simulink model "c00011M_harness"  (R2018a)
settings: Solver=FixedStepAuto  StartTime=0.0  StopTime=300  FixedStep=0.1  RelTol=1e-3
undefined symbols (not defined in the file): A1, hmax, PriorityTank, R1, R2, sigbuilder_block
(part 72 of 73)

== stateflow chart c00011M_harness/M160/Tank1/Control/Maintenance/Chart ==
  state InitialState
    entry: LiquidIn = 0;
    LiquidOut = 0;
  state Step1
    entry: LiquidIn = 0;
    LiquidOut = 1;
  state Step2
    entry: LiquidIn = 1;
    LiquidOut = 0;
  state Step3
    entry: LiquidIn = 0;
    LiquidOut = 1;
  (default) -> InitialState
  Step3 -> InitialState : [Type~=1||LiquidLevel <=0.01]
  Step2 -> InitialState [order 1] : [Type~=1]
  Step1 -> InitialState [order 1] : [Type ~= 1]
  InitialState -> Step1 : [StartMaintenance == 1 && Type ==1]
  Step1 -> Step2 [order 2] : [LiquidLevel <=0.01]
  Step2 -> Step3 [order 2] : [LiquidLevel>=hmax*0.9]
  data: Type input; StartMaintenance input; LiquidIn output; LiquidOut output; LiquidLevel input; hmax parameter

== stateflow chart c00011M_harness/M160/Tank2/Control/Maintenance/Chart ==
  state InitialState
    entry: LiquidIn = 0;
    LiquidOut = 0;
  state Step1
    entry: LiquidIn = 0;
    LiquidOut = 1;
  state Step2
    entry: LiquidIn = 1;
    LiquidOut = 0;
  state Step3
    entry: LiquidIn = 0;
    LiquidOut = 1;
  (default) -> InitialState
  Step3 -> InitialState : [Type~=1||LiquidLevel <=0.01]
  Step2 -> InitialState [order 1] : [Type~=1]
  Step1 -> InitialState [order 1] : [Type ~= 1]
  InitialState -> Step1 : [StartMaintenance == 1 && Type ==1]
  Step1 -> Step2 [order 2] : [LiquidLevel <=0.01]
  Step2 -> Step3 [order 2] : [LiquidLevel>=hmax*0.9]
  data: Type input; StartMaintenance input; LiquidIn output; LiquidOut output; LiquidLevel input; hmax parameter

== stateflow chart c00011M_harness/M161/Tank1/Control/Maintenance/Chart ==
  state InitialState
    entry: LiquidIn = 0;
    LiquidOut = 0;
  state Step1
    entry: LiquidIn = 0;
    LiquidOut = 1;
  state Step2
    entry: LiquidIn = 1;
    LiquidOut = 0;
  state Step3
    entry: LiquidIn = 0;
    LiquidOut = 1;
  (default) -> InitialState
  Step3 -> InitialState : [Type~=1||LiquidLevel <=0.01]
  Step2 -> InitialState [order 1] : [Type~=1]
  Step1 -> InitialState [order 1] : [Type ~= 1]
  InitialState -> Step1 : [StartMaintenance == 1 && Type ==1]
  Step1 -> Step2 [order 2] : [LiquidLevel <=0.01]
  Step2 -> Step3 [order 2] : [LiquidLevel>=hmax*0.9]
  data: Type input; StartMaintenance input; LiquidIn output; LiquidOut output; LiquidLevel input; hmax parameter

== stateflow chart c00011M_harness/M161/Tank2/Control/Maintenance/Chart ==
  state InitialState
    entry: LiquidIn = 0;
    LiquidOut = 0;
  state Step1
    entry: LiquidIn = 0;
    LiquidOut = 1;
  state Step2
    entry: LiquidIn = 1;
    LiquidOut = 0;
  state Step3
    entry: LiquidIn = 0;
    LiquidOut = 1;
  (default) -> InitialState
  Step3 -> InitialState : [Type~=1||LiquidLevel <=0.01]
  Step2 -> InitialState [order 1] : [Type~=1]
  Step1 -> InitialState [order 1] : [Type ~= 1]
  InitialState -> Step1 : [StartMaintenance == 1 && Type ==1]
  Step1 -> Step2 [order 2] : [LiquidLevel <=0.01]
  Step2 -> Step3 [order 2] : [LiquidLevel>=hmax*0.9]
  data: Type input; StartMaintenance input; LiquidIn output; LiquidOut output; LiquidLevel input; hmax parameter

== stateflow chart c00011M_harness/M162/Tank1/Control/Maintenance/Chart ==
  state InitialState
    entry: LiquidIn = 0;
    LiquidOut = 0;
  state Step1
    entry: LiquidIn = 0;
    LiquidOut = 1;
  state Step2
    entry: LiquidIn = 1;
    LiquidOut = 0;
  state Step3
    entry: LiquidIn = 0;
    LiquidOut = 1;
  (default) -> InitialState
  Step3 -> InitialState : [Type~=1||LiquidLevel <=0.01]
  Step2 -> InitialState [order 1] : [Type~=1]
  Step1 -> InitialState [order 1] : [Type ~= 1]
  InitialState -> Step1 : [StartMaintenance == 1 && Type ==1]
  Step1 -> Step2 [order 2] : [LiquidLevel <=0.01]
  Step2 -> Step3 [order 2] : [LiquidLevel>=hmax*0.9]
  data: Type input; StartMaintenance input; LiquidIn output; LiquidOut output; LiquidLevel input; hmax parameter

== stateflow chart c00011M_harness/M162/Tank2/Control/Maintenance/Chart ==
  state InitialState
    entry: LiquidIn = 0;
    LiquidOut = 0;
  state Step1
    entry: LiquidIn = 0;
    LiquidOut = 1;
  state Step2
    entry: LiquidIn = 1;
    LiquidOut = 0;
  state Step3
    entry: LiquidIn = 0;
    LiquidOut = 1;
  (default) -> InitialState
  Step3 -> InitialState : [Type~=1||LiquidLevel <=0.01]
  Step2 -> InitialState [order 1] : [Type~=1]
  Step1 -> InitialState [order 1] : [Type ~= 1]
  InitialState -> Step1 : [StartMaintenance == 1 && Type ==1]
  Step1 -> Step2 [order 2] : [LiquidLevel <=0.01]
  Step2 -> Step3 [order 2] : [LiquidLevel>=hmax*0.9]
  data: Type input; StartMaintenance input; LiquidIn output; LiquidOut output; LiquidLevel input; hmax parameter

== stateflow chart c00011M_harness/M163/Tank1/Control/Maintenance/Chart ==
  state InitialState
    entry: LiquidIn = 0;
    LiquidOut = 0;
  state Step1
    entry: LiquidIn = 0;
    LiquidOut = 1;
  state Step2
    entry: LiquidIn = 1;
    LiquidOut = 0;
  state Step3
    entry: LiquidIn = 0;
    LiquidOut = 1;
  (default) -> InitialState
  Step3 -> InitialState : [Type~=1||LiquidLevel <=0.01]
  Step2 -> InitialState [order 1] : [Type~=1]
  Step1 -> InitialState [order 1] : [Type ~= 1]
  InitialState -> Step1 : [StartMaintenance == 1 && Type ==1]
  Step1 -> Step2 [order 2] : [LiquidLevel <=0.01]
  Step2 -> Step3 [order 2] : [LiquidLevel>=hmax*0.9]
  data: Type input; StartMaintenance input; LiquidIn output; LiquidOut output; LiquidLevel input; hmax parameter

== stateflow chart c00011M_harness/M163/Tank2/Control/Maintenance/Chart ==
  state InitialState
    entry: LiquidIn = 0;
    LiquidOut = 0;
  state Step1
    entry: LiquidIn = 0;
    LiquidOut = 1;
  state Step2
    entry: LiquidIn = 1;
    LiquidOut = 0;
  state Step3
    entry: LiquidIn = 0;
    LiquidOut = 1;
  (default) -> InitialState
  Step3 -> InitialState : [Type~=1||LiquidLevel <=0.01]
  Step2 -> InitialState [order 1] : [Type~=1]
  Step1 -> InitialState [order 1] : [Type ~= 1]
  InitialState -> Step1 : [StartMaintenance == 1 && Type ==1]
  Step1 -> Step2 [order 2] : [LiquidLevel <=0.01]
  Step2 -> Step3 [order 2] : [LiquidLevel>=hmax*0.9]
  data: Type input; StartMaintenance input; LiquidIn output; LiquidOut output; LiquidLevel input; hmax parameter

== stateflow chart c00011M_harness/M164/Tank1/Control/Maintenance/Chart ==
  state InitialState
    entry: LiquidIn = 0;
    LiquidOut = 0;
  state Step1
    entry: LiquidIn = 0;
    LiquidOut = 1;
  state Step2
    entry: LiquidIn = 1;
    LiquidOut = 0;
  state Step3
    entry: LiquidIn = 0;
    LiquidOut = 1;
  (default) -> InitialState
  Step3 -> InitialState : [Type~=1||LiquidLevel <=0.01]
  Step2 -> InitialState [order 1] : [Type~=1]
  Step1 -> InitialState [order 1] : [Type ~= 1]
  InitialState -> Step1 : [StartMaintenance == 1 && Type ==1]
  Step1 -> Step2 [order 2] : [LiquidLevel <=0.01]
  Step2 -> Step3 [order 2] : [LiquidLevel>=hmax*0.9]
  data: Type input; StartMaintenance input; LiquidIn output; LiquidOut output; LiquidLevel input; hmax parameter

== stateflow chart c00011M_harness/M164/Tank2/Control/Maintenance/Chart ==
  state InitialState
    entry: LiquidIn = 0;
    LiquidOut = 0;
  state Step1
    entry: LiquidIn = 0;
    LiquidOut = 1;
  state Step2
    entry: LiquidIn = 1;
    LiquidOut = 0;
  state Step3
    entry: LiquidIn = 0;
    LiquidOut = 1;
  (default) -> InitialState
  Step3 -> InitialState : [Type~=1||LiquidLevel <=0.01]
  Step2 -> InitialState [order 1] : [Type~=1]
  Step1 -> InitialState [order 1] : [Type ~= 1]
  InitialState -> Step1 : [StartMaintenance == 1 && Type ==1]
  Step1 -> Step2 [order 2] : [LiquidLevel <=0.01]
  Step2 -> Step3 [order 2] : [LiquidLevel>=hmax*0.9]
  data: Type input; StartMaintenance input; LiquidIn output; LiquidOut output; LiquidLevel input; hmax parameter

== stateflow chart c00011M_harness/M165/Tank1/Control/Maintenance/Chart ==
  state InitialState
    entry: LiquidIn = 0;
    LiquidOut = 0;
  state Step1
    entry: LiquidIn = 0;
    LiquidOut = 1;
  state Step2
    entry: LiquidIn = 1;
    LiquidOut = 0;
  state Step3
    entry: LiquidIn = 0;
    LiquidOut = 1;
  (default) -> InitialState
  Step3 -> InitialState : [Type~=1||LiquidLevel <=0.01]
  Step2 -> InitialState [order 1] : [Type~=1]
  Step1 -> InitialState [order 1] : [Type ~= 1]
  InitialState -> Step1 : [StartMaintenance == 1 && Type ==1]
  Step1 -> Step2 [order 2] : [LiquidLevel <=0.01]
  Step2 -> Step3 [order 2] : [LiquidLevel>=hmax*0.9]
  data: Type input; StartMaintenance input; LiquidIn output; LiquidOut output; LiquidLevel input; hmax parameter

== stateflow chart c00011M_harness/M165/Tank2/Control/Maintenance/Chart ==
  state InitialState
    entry: LiquidIn = 0;
    LiquidOut = 0;
  state Step1
    entry: LiquidIn = 0;
    LiquidOut = 1;
  state Step2
    entry: LiquidIn = 1;
    LiquidOut = 0;
  state Step3
    entry: LiquidIn = 0;
    LiquidOut = 1;
  (default) -> InitialState
  Step3 -> InitialState : [Type~=1||LiquidLevel <=0.01]
  Step2 -> InitialState [order 1] : [Type~=1]
  Step1 -> InitialState [order 1] : [Type ~= 1]
  InitialState -> Step1 : [StartMaintenance == 1 && Type ==1]
  Step1 -> Step2 [order 2] : [LiquidLevel <=0.01]
  Step2 -> Step3 [order 2] : [LiquidLevel>=hmax*0.9]
  data: Type input; StartMaintenance input; LiquidIn output; LiquidOut output; LiquidLevel input; hmax parameter

== stateflow chart c00011M_harness/M200/Tank1/Control/Maintenance/Chart ==
  state InitialState
    entry: LiquidIn = 0;
    LiquidOut = 0;
  state Step1
    entry: LiquidIn = 0;
    LiquidOut = 1;
  state Step2
    entry: LiquidIn = 1;
    LiquidOut = 0;
  state Step3
    entry: LiquidIn = 0;
    LiquidOut = 1;
  (default) -> InitialState
  Step3 -> InitialState : [Type~=1||LiquidLevel <=0.01]
  Step2 -> InitialState [order 1] : [Type~=1]
  Step1 -> InitialState [order 1] : [Type ~= 1]
  InitialState -> Step1 : [StartMaintenance == 1 && Type ==1]
  Step1 -> Step2 [order 2] : [LiquidLevel <=0.01]
  Step2 -> Step3 [order 2] : [LiquidLevel>=hmax*0.9]
  data: Type input; StartMaintenance input; LiquidIn output; LiquidOut output; LiquidLevel input; hmax parameter

== stateflow chart c00011M_harness/M200/Tank2/Control/Maintenance/Chart ==
  state InitialState
    entry: LiquidIn = 0;
    LiquidOut = 0;
  state Step1
    entry: LiquidIn = 0;
    LiquidOut = 1;
  state Step2
    entry: LiquidIn = 1;
    LiquidOut = 0;
  state Step3
    entry: LiquidIn = 0;
    LiquidOut = 1;
  (default) -> InitialState
  Step3 -> InitialState : [Type~=1||LiquidLevel <=0.01]
  Step2 -> InitialState [order 1] : [Type~=1]
  Step1 -> InitialState [order 1] : [Type ~= 1]
  InitialState -> Step1 : [StartMaintenance == 1 && Type ==1]
  Step1 -> Step2 [order 2] : [LiquidLevel <=0.01]
  Step2 -> Step3 [order 2] : [LiquidLevel>=hmax*0.9]
  data: Type input; StartMaintenance input; LiquidIn output; LiquidOut output; LiquidLevel input; hmax parameter

== stateflow chart c00011M_harness/M201/Tank1/Control/Maintenance/Chart ==
  state InitialState
    entry: LiquidIn = 0;
    LiquidOut = 0;
  state Step1
    entry: LiquidIn = 0;
    LiquidOut = 1;
  state Step2
    entry: LiquidIn = 1;
    LiquidOut = 0;
  state Step3
    entry: LiquidIn = 0;
    LiquidOut = 1;
  (default) -> InitialState
  Step3 -> InitialState : [Type~=1||LiquidLevel <=0.01]
  Step2 -> InitialState [order 1] : [Type~=1]
  Step1 -> InitialState [order 1] : [Type ~= 1]
  InitialState -> Step1 : [StartMaintenance == 1 && Type ==1]
  Step1 -> Step2 [order 2] : [LiquidLevel <=0.01]
  Step2 -> Step3 [order 2] : [LiquidLevel>=hmax*0.9]
  data: Type input; StartMaintenance input; LiquidIn output; LiquidOut output; LiquidLevel input; hmax parameter

== stateflow chart c00011M_harness/M201/Tank2/Control/Maintenance/Chart ==
  state InitialState
    entry: LiquidIn = 0;
    LiquidOut = 0;
  state Step1
    entry: LiquidIn = 0;
    LiquidOut = 1;
  state Step2
    entry: LiquidIn = 1;
    LiquidOut = 0;
  state Step3
    entry: LiquidIn = 0;
    LiquidOut = 1;
  (default) -> InitialState
  Step3 -> InitialState : [Type~=1||LiquidLevel <=0.01]
  Step2 -> InitialState [order 1] : [Type~=1]
  Step1 -> InitialState [order 1] : [Type ~= 1]
  InitialState -> Step1 : [StartMaintenance == 1 && Type ==1]
  Step1 -> Step2 [order 2] : [LiquidLevel <=0.01]
  Step2 -> Step3 [order 2] : [LiquidLevel>=hmax*0.9]
  data: Type input; StartMaintenance input; LiquidIn output; LiquidOut output; LiquidLevel input; hmax parameter

== stateflow chart c00011M_harness/M202/Tank1/Control/Maintenance/Chart ==
  state InitialState
    entry: LiquidIn = 0;
    LiquidOut = 0;
  state Step1
    entry: LiquidIn = 0;
    LiquidOut = 1;
  state Step2
    entry: LiquidIn = 1;
    LiquidOut = 0;
  state Step3
    entry: LiquidIn = 0;
    LiquidOut = 1;
  (default) -> InitialState
  Step3 -> InitialState : [Type~=1||LiquidLevel <=0.01]
  Step2 -> InitialState [order 1] : [Type~=1]
  Step1 -> InitialState [order 1] : [Type ~= 1]
  InitialState -> Step1 : [StartMaintenance == 1 && Type ==1]
  Step1 -> Step2 [order 2] : [LiquidLevel <=0.01]
  Step2 -> Step3 [order 2] : [LiquidLevel>=hmax*0.9]
  data: Type input; StartMaintenance input; LiquidIn output; LiquidOut output; LiquidLevel input; hmax parameter

== stateflow chart c00011M_harness/M202/Tank2/Control/Maintenance/Chart ==
  state InitialState
    entry: LiquidIn = 0;
    LiquidOut = 0;
  state Step1
    entry: LiquidIn = 0;
    LiquidOut = 1;
  state Step2
    entry: LiquidIn = 1;
    LiquidOut = 0;
  state Step3
    entry: LiquidIn = 0;
    LiquidOut = 1;
  (default) -> InitialState
  Step3 -> InitialState : [Type~=1||LiquidLevel <=0.01]
  Step2 -> InitialState [order 1] : [Type~=1]
  Step1 -> InitialState [order 1] : [Type ~= 1]
  InitialState -> Step1 : [StartMaintenance == 1 && Type ==1]
  Step1 -> Step2 [order 2] : [LiquidLevel <=0.01]
  Step2 -> Step3 [order 2] : [LiquidLevel>=hmax*0.9]
  data: Type input; StartMaintenance input; LiquidIn output; LiquidOut output; LiquidLevel input; hmax parameter

== stateflow chart c00011M_harness/M203/Tank1/Control/Maintenance/Chart ==
  state InitialState
    entry: LiquidIn = 0;
    LiquidOut = 0;
  state Step1
    entry: LiquidIn = 0;
    LiquidOut = 1;
  state Step2
    entry: LiquidIn = 1;
    LiquidOut = 0;
  state Step3
    entry: LiquidIn = 0;
    LiquidOut = 1;
  (default) -> InitialState
  Step3 -> InitialState : [Type~=1||LiquidLevel <=0.01]
  Step2 -> InitialState [order 1] : [Type~=1]
  Step1 -> InitialState [order 1] : [Type ~= 1]
  InitialState -> Step1 : [StartMaintenance == 1 && Type ==1]
  Step1 -> Step2 [order 2] : [LiquidLevel <=0.01]
  Step2 -> Step3 [order 2] : [LiquidLevel>=hmax*0.9]
  data: Type input; StartMaintenance input; LiquidIn output; LiquidOut output; LiquidLevel input; hmax parameter

== stateflow chart c00011M_harness/M203/Tank2/Control/Maintenance/Chart ==
  state InitialState
    entry: LiquidIn = 0;
    LiquidOut = 0;
  state Step1
    entry: LiquidIn = 0;
    LiquidOut = 1;
  state Step2
    entry: LiquidIn = 1;
    LiquidOut = 0;
  state Step3
    entry: LiquidIn = 0;
    LiquidOut = 1;
  (default) -> InitialState
  Step3 -> InitialState : [Type~=1||LiquidLevel <=0.01]
  Step2 -> InitialState [order 1] : [Type~=1]
  Step1 -> InitialState [order 1] : [Type ~= 1]
  InitialState -> Step1 : [StartMaintenance == 1 && Type ==1]
  Step1 -> Step2 [order 2] : [LiquidLevel <=0.01]
  Step2 -> Step3 [order 2] : [LiquidLevel>=hmax*0.9]
  data: Type input; StartMaintenance input; LiquidIn output; LiquidOut output; LiquidLevel input; hmax parameter

== stateflow chart c00011M_harness/M204/Tank1/Control/Maintenance/Chart ==
  state InitialState
    entry: LiquidIn = 0;
    LiquidOut = 0;
  state Step1
    entry: LiquidIn = 0;
    LiquidOut = 1;
  state Step2
    entry: LiquidIn = 1;
    LiquidOut = 0;
  state Step3
    entry: LiquidIn = 0;
    LiquidOut = 1;
  (default) -> InitialState
  Step3 -> InitialState : [Type~=1||LiquidLevel <=0.01]
  Step2 -> InitialState [order 1] : [Type~=1]
  Step1 -> InitialState [order 1] : [Type ~= 1]
  InitialState -> Step1 : [StartMaintenance == 1 && Type ==1]
  Step1 -> Step2 [order 2] : [LiquidLevel <=0.01]
  Step2 -> Step3 [order 2] : [LiquidLevel>=hmax*0.9]
  data: Type input; StartMaintenance input; LiquidIn output; LiquidOut output; LiquidLevel input; hmax parameter

== stateflow chart c00011M_harness/M204/Tank2/Control/Maintenance/Chart ==
  state InitialState
    entry: LiquidIn = 0;
    LiquidOut = 0;
  state Step1
    entry: LiquidIn = 0;
    LiquidOut = 1;
  state Step2
    entry: LiquidIn = 1;
    LiquidOut = 0;
  state Step3
    entry: LiquidIn = 0;
    LiquidOut = 1;
  (default) -> InitialState
  Step3 -> InitialState : [Type~=1||LiquidLevel <=0.01]
  Step2 -> InitialState [order 1] : [Type~=1]
  Step1 -> InitialState [order 1] : [Type ~= 1]
  InitialState -> Step1 : [StartMaintenance == 1 && Type ==1]
  Step1 -> Step2 [order 2] : [LiquidLevel <=0.01]
  Step2 -> Step3 [order 2] : [LiquidLevel>=hmax*0.9]
  data: Type input; StartMaintenance input; LiquidIn output; LiquidOut output; LiquidLevel input; hmax parameter

== stateflow chart c00011M_harness/M205/Tank1/Control/Maintenance/Chart ==
  state InitialState
    entry: LiquidIn = 0;
    LiquidOut = 0;
  state Step1
    entry: LiquidIn = 0;
    LiquidOut = 1;
  state Step2
    entry: LiquidIn = 1;
    LiquidOut = 0;
  state Step3
    entry: LiquidIn = 0;
    LiquidOut = 1;
  (default) -> InitialState
  Step3 -> InitialState : [Type~=1||LiquidLevel <=0.01]
  Step2 -> InitialState [order 1] : [Type~=1]
  Step1 -> InitialState [order 1] : [Type ~= 1]
  InitialState -> Step1 : [StartMaintenance == 1 && Type ==1]
  Step1 -> Step2 [order 2] : [LiquidLevel <=0.01]
  Step2 -> Step3 [order 2] : [LiquidLevel>=hmax*0.9]
  data: Type input; StartMaintenance input; LiquidIn output; LiquidOut output; LiquidLevel input; hmax parameter

== stateflow chart c00011M_harness/M205/Tank2/Control/Maintenance/Chart ==
  state InitialState
    entry: LiquidIn = 0;
    LiquidOut = 0;
  state Step1
    entry: LiquidIn = 0;
    LiquidOut = 1;
  state Step2
    entry: LiquidIn = 1;
    LiquidOut = 0;
  state Step3
    entry: LiquidIn = 0;
    LiquidOut = 1;
  (default) -> InitialState
  Step3 -> InitialState : [Type~=1||LiquidLevel <=0.01]
  Step2 -> InitialState [order 1] : [Type~=1]
  Step1 -> InitialState [order 1] : [Type ~= 1]
  InitialState -> Step1 : [StartMaintenance == 1 && Type ==1]
  Step1 -> Step2 [order 2] : [LiquidLevel <=0.01]
  Step2 -> Step3 [order 2] : [LiquidLevel>=hmax*0.9]
  data: Type input; StartMaintenance input; LiquidIn output; LiquidOut output; LiquidLevel input; hmax parameter

== stateflow chart c00011M_harness/M206/Tank1/Control/Maintenance/Chart ==
  state InitialState
    entry: LiquidIn = 0;
    LiquidOut = 0;
  state Step1
    entry: LiquidIn = 0;
    LiquidOut = 1;
  state Step2
    entry: LiquidIn = 1;
    LiquidOut = 0;
  state Step3
    entry: LiquidIn = 0;
    LiquidOut = 1;
  (default) -> InitialState
  Step3 -> InitialState : [Type~=1||LiquidLevel <=0.01]
  Step2 -> InitialState [order 1] : [Type~=1]
  Step1 -> InitialState [order 1] : [Type ~= 1]
  InitialState -> Step1 : [StartMaintenance == 1 && Type ==1]
  Step1 -> Step2 [order 2] : [LiquidLevel <=0.01]
  Step2 -> Step3 [order 2] : [LiquidLevel>=hmax*0.9]
  data: Type input; StartMaintenance input; LiquidIn output; LiquidOut output; LiquidLevel input; hmax parameter

== stateflow chart c00011M_harness/M206/Tank2/Control/Maintenance/Chart ==
  state InitialState
    entry: LiquidIn = 0;
    LiquidOut = 0;
  state Step1
    entry: LiquidIn = 0;
    LiquidOut = 1;
  state Step2
    entry: LiquidIn = 1;
    LiquidOut = 0;
  state Step3
    entry: LiquidIn = 0;
    LiquidOut = 1;
  (default) -> InitialState
  Step3 -> InitialState : [Type~=1||LiquidLevel <=0.01]
  Step2 -> InitialState [order 1] : [Type~=1]
  Step1 -> InitialState [order 1] : [Type ~= 1]
  InitialState -> Step1 : [StartMaintenance == 1 && Type ==1]
  Step1 -> Step2 [order 2] : [LiquidLevel <=0.01]
  Step2 -> Step3 [order 2] : [LiquidLevel>=hmax*0.9]
  data: Type input; StartMaintenance input; LiquidIn output; LiquidOut output; LiquidLevel input; hmax parameter

== stateflow chart c00011M_harness/M207/Tank1/Control/Maintenance/Chart ==
  state InitialState
    entry: LiquidIn = 0;
    LiquidOut = 0;
  state Step1
    entry: LiquidIn = 0;
    LiquidOut = 1;
  state Step2
    entry: LiquidIn = 1;
    LiquidOut = 0;
  state Step3
    entry: LiquidIn = 0;
    LiquidOut = 1;
  (default) -> InitialState
  Step3 -> InitialState : [Type~=1||LiquidLevel <=0.01]
  Step2 -> InitialState [order 1] : [Type~=1]
  Step1 -> InitialState [order 1] : [Type ~= 1]
  InitialState -> Step1 : [StartMaintenance == 1 && Type ==1]
  Step1 -> Step2 [order 2] : [LiquidLevel <=0.01]
  Step2 -> Step3 [order 2] : [LiquidLevel>=hmax*0.9]
  data: Type input; StartMaintenance input; LiquidIn output; LiquidOut output; LiquidLevel input; hmax parameter

== stateflow chart c00011M_harness/M207/Tank2/Control/Maintenance/Chart ==
  state InitialState
    entry: LiquidIn = 0;
    LiquidOut = 0;
  state Step1
    entry: LiquidIn = 0;
    LiquidOut = 1;
  state Step2
    entry: LiquidIn = 1;
    LiquidOut = 0;
  state Step3
    entry: LiquidIn = 0;
    LiquidOut = 1;
  (default) -> InitialState
  Step3 -> InitialState : [Type~=1||LiquidLevel <=0.01]
  Step2 -> InitialState [order 1] : [Type~=1]
  Step1 -> InitialState [order 1] : [Type ~= 1]
  InitialState -> Step1 : [StartMaintenance == 1 && Type ==1]
  Step1 -> Step2 [order 2] : [LiquidLevel <=0.01]
  Step2 -> Step3 [order 2] : [LiquidLevel>=hmax*0.9]
  data: Type input; StartMaintenance input; LiquidIn output; LiquidOut output; LiquidLevel input; hmax parameter

== stateflow chart c00011M_harness/M208/Tank1/Control/Maintenance/Chart ==
  state InitialState
    entry: LiquidIn = 0;
    LiquidOut = 0;
  state Step1
    entry: LiquidIn = 0;
    LiquidOut = 1;
  state Step2
    entry: LiquidIn = 1;
    LiquidOut = 0;
  state Step3
    entry: LiquidIn = 0;
    LiquidOut = 1;
  (default) -> InitialState
  Step3 -> InitialState : [Type~=1||LiquidLevel <=0.01]
  Step2 -> InitialState [order 1] : [Type~=1]
  Step1 -> InitialState [order 1] : [Type ~= 1]
  InitialState -> Step1 : [StartMaintenance == 1 && Type ==1]
  Step1 -> Step2 [order 2] : [LiquidLevel <=0.01]
  Step2 -> Step3 [order 2] : [LiquidLevel>=hmax*0.9]
  data: Type input; StartMaintenance input; LiquidIn output; LiquidOut output; LiquidLevel input; hmax parameter

== stateflow chart c00011M_harness/M208/Tank2/Control/Maintenance/Chart ==
  state InitialState
    entry: LiquidIn = 0;
    LiquidOut = 0;
  state Step1
    entry: LiquidIn = 0;
    LiquidOut = 1;
  state Step2
    entry: LiquidIn = 1;
    LiquidOut = 0;
  state Step3
    entry: LiquidIn = 0;
    LiquidOut = 1;
  (default) -> InitialState
  Step3 -> InitialState : [Type~=1||LiquidLevel <=0.01]
  Step2 -> InitialState [order 1] : [Type~=1]
  Step1 -> InitialState [order 1] : [Type ~= 1]
  InitialState -> Step1 : [StartMaintenance == 1 && Type ==1]
  Step1 -> Step2 [order 2] : [LiquidLevel <=0.01]
  Step2 -> Step3 [order 2] : [LiquidLevel>=hmax*0.9]
  data: Type input; StartMaintenance input; LiquidIn output; LiquidOut output; LiquidLevel input; hmax parameter

== stateflow chart c00011M_harness/M209/Tank1/Control/Maintenance/Chart ==
  state InitialState
    entry: LiquidIn = 0;
    LiquidOut = 0;
  state Step1
    entry: LiquidIn = 0;
    LiquidOut = 1;
  state Step2
    entry: LiquidIn = 1;
    LiquidOut = 0;
  state Step3
    entry: LiquidIn = 0;
    LiquidOut = 1;
  (default) -> InitialState
  Step3 -> InitialState : [Type~=1||LiquidLevel <=0.01]
  Step2 -> InitialState [order 1] : [Type~=1]
  Step1 -> InitialState [order 1] : [Type ~= 1]
  InitialState -> Step1 : [StartMaintenance == 1 && Type ==1]
  Step1 -> Step2 [order 2] : [LiquidLevel <=0.01]
  Step2 -> Step3 [order 2] : [LiquidLevel>=hmax*0.9]
  data: Type input; StartMaintenance input; LiquidIn output; LiquidOut output; LiquidLevel input; hmax parameter

== stateflow chart c00011M_harness/M209/Tank2/Control/Maintenance/Chart ==
  state InitialState
    entry: LiquidIn = 0;
    LiquidOut = 0;
  state Step1
    entry: LiquidIn = 0;
    LiquidOut = 1;
  state Step2
    entry: LiquidIn = 1;
    LiquidOut = 0;
  state Step3
    entry: LiquidIn = 0;
    LiquidOut = 1;
  (default) -> InitialState
  Step3 -> InitialState : [Type~=1||LiquidLevel <=0.01]
  Step2 -> InitialState [order 1] : [Type~=1]
  Step1 -> InitialState [order 1] : [Type ~= 1]
  InitialState -> Step1 : [StartMaintenance == 1 && Type ==1]
  Step1 -> Step2 [order 2] : [LiquidLevel <=0.01]
  Step2 -> Step3 [order 2] : [LiquidLevel>=hmax*0.9]
  data: Type input; StartMaintenance input; LiquidIn output; LiquidOut output; LiquidLevel input; hmax parameter

== stateflow chart c00011M_harness/M222/Tank1/Control/Maintenance/Chart ==
  state InitialState
    entry: LiquidIn = 0;
    LiquidOut = 0;
  state Step1
    entry: LiquidIn = 0;
    LiquidOut = 1;
  state Step2
    entry: LiquidIn = 1;
    LiquidOut = 0;
  state Step3
    entry: LiquidIn = 0;
    LiquidOut = 1;
  (default) -> InitialState
  Step3 -> InitialState : [Type~=1||LiquidLevel <=0.01]
  Step2 -> InitialState [order 1] : [Type~=1]
  Step1 -> InitialState [order 1] : [Type ~= 1]
  InitialState -> Step1 : [StartMaintenance == 1 && Type ==1]
  Step1 -> Step2 [order 2] : [LiquidLevel <=0.01]
  Step2 -> Step3 [order 2] : [LiquidLevel>=hmax*0.9]
  data: Type input; StartMaintenance input; LiquidIn output; LiquidOut output; LiquidLevel input; hmax parameter

== stateflow chart c00011M_harness/M222/Tank2/Control/Maintenance/Chart ==
  state InitialState
    entry: LiquidIn = 0;
    LiquidOut = 0;
  state Step1
    entry: LiquidIn = 0;
    LiquidOut = 1;
  state Step2
    entry: LiquidIn = 1;
    LiquidOut = 0;
  state Step3
    entry: LiquidIn = 0;
    LiquidOut = 1;
  (default) -> InitialState
  Step3 -> InitialState : [Type~=1||LiquidLevel <=0.01]
  Step2 -> InitialState [order 1] : [Type~=1]
  Step1 -> InitialState [order 1] : [Type ~= 1]
  InitialState -> Step1 : [StartMaintenance == 1 && Type ==1]
  Step1 -> Step2 [order 2] : [LiquidLevel <=0.01]
  Step2 -> Step3 [order 2] : [LiquidLevel>=hmax*0.9]
  data: Type input; StartMaintenance input; LiquidIn output; LiquidOut output; LiquidLevel input; hmax parameter

== stateflow chart c00011M_harness/M223/Tank1/Control/Maintenance/Chart ==
  state InitialState
    entry: LiquidIn = 0;
    LiquidOut = 0;
  state Step1
    entry: LiquidIn = 0;
    LiquidOut = 1;
  state Step2
    entry: LiquidIn = 1;
    LiquidOut = 0;
  state Step3
    entry: LiquidIn = 0;
    LiquidOut = 1;
  (default) -> InitialState
  Step3 -> InitialState : [Type~=1||LiquidLevel <=0.01]
  Step2 -> InitialState [order 1] : [Type~=1]
  Step1 -> InitialState [order 1] : [Type ~= 1]
  InitialState -> Step1 : [StartMaintenance == 1 && Type ==1]
  Step1 -> Step2 [order 2] : [LiquidLevel <=0.01]
  Step2 -> Step3 [order 2] : [LiquidLevel>=hmax*0.9]
  data: Type input; StartMaintenance input; LiquidIn output; LiquidOut output; LiquidLevel input; hmax parameter

== stateflow chart c00011M_harness/M223/Tank2/Control/Maintenance/Chart ==
  state InitialState
    entry: LiquidIn = 0;
    LiquidOut = 0;
  state Step1
    entry: LiquidIn = 0;
    LiquidOut = 1;
  state Step2
    entry: LiquidIn = 1;
    LiquidOut = 0;
  state Step3
    entry: LiquidIn = 0;
    LiquidOut = 1;
  (default) -> InitialState
  Step3 -> InitialState : [Type~=1||LiquidLevel <=0.01]
  Step2 -> InitialState [order 1] : [Type~=1]
  Step1 -> InitialState [order 1] : [Type ~= 1]
  InitialState -> Step1 : [StartMaintenance == 1 && Type ==1]
  Step1 -> Step2 [order 2] : [LiquidLevel <=0.01]
  Step2 -> Step3 [order 2] : [LiquidLevel>=hmax*0.9]
  data: Type input; StartMaintenance input; LiquidIn output; LiquidOut output; LiquidLevel input; hmax parameter

== stateflow chart c00011M_harness/M224/Tank1/Control/Maintenance/Chart ==
  state InitialState
    entry: LiquidIn = 0;
    LiquidOut = 0;
  state Step1
    entry: LiquidIn = 0;
    LiquidOut = 1;
  state Step2
    entry: LiquidIn = 1;
    LiquidOut = 0;
  state Step3
    entry: LiquidIn = 0;
    LiquidOut = 1;
  (default) -> InitialState
  Step3 -> InitialState : [Type~=1||LiquidLevel <=0.01]
  Step2 -> InitialState [order 1] : [Type~=1]
  Step1 -> InitialState [order 1] : [Type ~= 1]
  InitialState -> Step1 : [StartMaintenance == 1 && Type ==1]
  Step1 -> Step2 [order 2] : [LiquidLevel <=0.01]
  Step2 -> Step3 [order 2] : [LiquidLevel>=hmax*0.9]
  data: Type input; StartMaintenance input; LiquidIn output; LiquidOut output; LiquidLevel input; hmax parameter

== stateflow chart c00011M_harness/M224/Tank2/Control/Maintenance/Chart ==
  state InitialState
    entry: LiquidIn = 0;
    LiquidOut = 0;
  state Step1
    entry: LiquidIn = 0;
    LiquidOut = 1;
  state Step2
    entry: LiquidIn = 1;
    LiquidOut = 0;
  state Step3
    entry: LiquidIn = 0;
    LiquidOut = 1;
  (default) -> InitialState
  Step3 -> InitialState : [Type~=1||LiquidLevel <=0.01]
  Step2 -> InitialState [order 1] : [Type~=1]
  Step1 -> InitialState [order 1] : [Type ~= 1]
  InitialState -> Step1 : [StartMaintenance == 1 && Type ==1]
  Step1 -> Step2 [order 2] : [LiquidLevel <=0.01]
  Step2 -> Step3 [order 2] : [LiquidLevel>=hmax*0.9]
  data: Type input; StartMaintenance input; LiquidIn output; LiquidOut output; LiquidLevel input; hmax parameter

== stateflow chart c00011M_harness/M225/Tank1/Control/Maintenance/Chart ==
  state InitialState
    entry: LiquidIn = 0;
    LiquidOut = 0;
  state Step1
    entry: LiquidIn = 0;
    LiquidOut = 1;
  state Step2
    entry: LiquidIn = 1;
    LiquidOut = 0;
  state Step3
    entry: LiquidIn = 0;
    LiquidOut = 1;
  (default) -> InitialState
  Step3 -> InitialState : [Type~=1||LiquidLevel <=0.01]
  Step2 -> InitialState [order 1] : [Type~=1]
  Step1 -> InitialState [order 1] : [Type ~= 1]
  InitialState -> Step1 : [StartMaintenance == 1 && Type ==1]
  Step1 -> Step2 [order 2] : [LiquidLevel <=0.01]
  Step2 -> Step3 [order 2] : [LiquidLevel>=hmax*0.9]
  data: Type input; StartMaintenance input; LiquidIn output; LiquidOut output; LiquidLevel input; hmax parameter

== stateflow chart c00011M_harness/M225/Tank2/Control/Maintenance/Chart ==
  state InitialState
    entry: LiquidIn = 0;
    LiquidOut = 0;
  state Step1
    entry: LiquidIn = 0;
    LiquidOut = 1;
  state Step2
    entry: LiquidIn = 1;
    LiquidOut = 0;
  state Step3
    entry: LiquidIn = 0;
    LiquidOut = 1;
  (default) -> InitialState
  Step3 -> InitialState : [Type~=1||LiquidLevel <=0.01]
  Step2 -> InitialState [order 1] : [Type~=1]
  Step1 -> InitialState [order 1] : [Type ~= 1]
  InitialState -> Step1 : [StartMaintenance == 1 && Type ==1]
  Step1 -> Step2 [order 2] : [LiquidLevel <=0.01]
  Step2 -> Step3 [order 2] : [LiquidLevel>=hmax*0.9]
  data: Type input; StartMaintenance input; LiquidIn output; LiquidOut output; LiquidLevel input; hmax parameter

== stateflow chart c00011M_harness/M226/Tank1/Control/Maintenance/Chart ==
  state InitialState
    entry: LiquidIn = 0;
    LiquidOut = 0;
  state Step1
    entry: LiquidIn = 0;
    LiquidOut = 1;
  state Step2
    entry: LiquidIn = 1;
    LiquidOut = 0;
  state Step3
    entry: LiquidIn = 0;
    LiquidOut = 1;
  (default) -> InitialState
  Step3 -> InitialState : [Type~=1||LiquidLevel <=0.01]
  Step2 -> InitialState [order 1] : [Type~=1]
  Step1 -> InitialState [order 1] : [Type ~= 1]
  InitialState -> Step1 : [StartMaintenance == 1 && Type ==1]
  Step1 -> Step2 [order 2] : [LiquidLevel <=0.01]
  Step2 -> Step3 [order 2] : [LiquidLevel>=hmax*0.9]
  data: Type input; StartMaintenance input; LiquidIn output; LiquidOut output; LiquidLevel input; hmax parameter

== stateflow chart c00011M_harness/M226/Tank2/Control/Maintenance/Chart ==
  state InitialState
    entry: LiquidIn = 0;
    LiquidOut = 0;
  state Step1
    entry: LiquidIn = 0;
    LiquidOut = 1;
  state Step2
    entry: LiquidIn = 1;
    LiquidOut = 0;
  state Step3
    entry: LiquidIn = 0;
    LiquidOut = 1;
  (default) -> InitialState
  Step3 -> InitialState : [Type~=1||LiquidLevel <=0.01]
  Step2 -> InitialState [order 1] : [Type~=1]
  Step1 -> InitialState [order 1] : [Type ~= 1]
  InitialState -> Step1 : [StartMaintenance == 1 && Type ==1]
  Step1 -> Step2 [order 2] : [LiquidLevel <=0.01]
  Step2 -> Step3 [order 2] : [LiquidLevel>=hmax*0.9]
  data: Type input; StartMaintenance input; LiquidIn output; LiquidOut output; LiquidLevel input; hmax parameter

== stateflow chart c00011M_harness/M227/Tank1/Control/Maintenance/Chart ==
  state InitialState
    entry: LiquidIn = 0;
    LiquidOut = 0;
  state Step1
    entry: LiquidIn = 0;
    LiquidOut = 1;
  state Step2
    entry: LiquidIn = 1;
    LiquidOut = 0;
  state Step3
    entry: LiquidIn = 0;
    LiquidOut = 1;
  (default) -> InitialState
  Step3 -> InitialState : [Type~=1||LiquidLevel <=0.01]
  Step2 -> InitialState [order 1] : [Type~=1]
  Step1 -> InitialState [order 1] : [Type ~= 1]
  InitialState -> Step1 : [StartMaintenance == 1 && Type ==1]
  Step1 -> Step2 [order 2] : [LiquidLevel <=0.01]
  Step2 -> Step3 [order 2] : [LiquidLevel>=hmax*0.9]
  data: Type input; StartMaintenance input; LiquidIn output; LiquidOut output; LiquidLevel input; hmax parameter

== stateflow chart c00011M_harness/M227/Tank2/Control/Maintenance/Chart ==
  state InitialState
    entry: LiquidIn = 0;
    LiquidOut = 0;
  state Step1
    entry: LiquidIn = 0;
    LiquidOut = 1;
  state Step2
    entry: LiquidIn = 1;
    LiquidOut = 0;
  state Step3
    entry: LiquidIn = 0;
    LiquidOut = 1;
  (default) -> InitialState
  Step3 -> InitialState : [Type~=1||LiquidLevel <=0.01]
  Step2 -> InitialState [order 1] : [Type~=1]
  Step1 -> InitialState [order 1] : [Type ~= 1]
  InitialState -> Step1 : [StartMaintenance == 1 && Type ==1]
  Step1 -> Step2 [order 2] : [LiquidLevel <=0.01]
  Step2 -> Step3 [order 2] : [LiquidLevel>=hmax*0.9]
  data: Type input; StartMaintenance input; LiquidIn output; LiquidOut output; LiquidLevel input; hmax parameter

== stateflow chart c00011M_harness/M228/Tank1/Control/Maintenance/Chart ==
  state InitialState
    entry: LiquidIn = 0;
    LiquidOut = 0;
  state Step1
    entry: LiquidIn = 0;
    LiquidOut = 1;
  state Step2
    entry: LiquidIn = 1;
    LiquidOut = 0;
  state Step3
    entry: LiquidIn = 0;
    LiquidOut = 1;
  (default) -> InitialState
  Step3 -> InitialState : [Type~=1||LiquidLevel <=0.01]
  Step2 -> InitialState [order 1] : [Type~=1]
  Step1 -> InitialState [order 1] : [Type ~= 1]
  InitialState -> Step1 : [StartMaintenance == 1 && Type ==1]
  Step1 -> Step2 [order 2] : [LiquidLevel <=0.01]
  Step2 -> Step3 [order 2] : [LiquidLevel>=hmax*0.9]
  data: Type input; StartMaintenance input; LiquidIn output; LiquidOut output; LiquidLevel input; hmax parameter

== stateflow chart c00011M_harness/M228/Tank2/Control/Maintenance/Chart ==
  state InitialState
    entry: LiquidIn = 0;
    LiquidOut = 0;
  state Step1
    entry: LiquidIn = 0;
    LiquidOut = 1;
  state Step2
    entry: LiquidIn = 1;
    LiquidOut = 0;
  state Step3
    entry: LiquidIn = 0;
    LiquidOut = 1;
  (default) -> InitialState
  Step3 -> InitialState : [Type~=1||LiquidLevel <=0.01]
  Step2 -> InitialState [order 1] : [Type~=1]
  Step1 -> InitialState [order 1] : [Type ~= 1]
  InitialState -> Step1 : [StartMaintenance == 1 && Type ==1]
  Step1 -> Step2 [order 2] : [LiquidLevel <=0.01]
  Step2 -> Step3 [order 2] : [LiquidLevel>=hmax*0.9]
  data: Type input; StartMaintenance input; LiquidIn output; LiquidOut output; LiquidLevel input; hmax parameter

== stateflow chart c00011M_harness/M229/Tank1/Control/Maintenance/Chart ==
  state InitialState
    entry: LiquidIn = 0;
    LiquidOut = 0;
  state Step1
    entry: LiquidIn = 0;
    LiquidOut = 1;
  state Step2
    entry: LiquidIn = 1;
    LiquidOut = 0;
  state Step3
    entry: LiquidIn = 0;
    LiquidOut = 1;
  (default) -> InitialState
  Step3 -> InitialState : [Type~=1||LiquidLevel <=0.01]
  Step2 -> InitialState [order 1] : [Type~=1]
  Step1 -> InitialState [order 1] : [Type ~= 1]
  InitialState -> Step1 : [StartMaintenance == 1 && Type ==1]
  Step1 -> Step2 [order 2] : [LiquidLevel <=0.01]
  Step2 -> Step3 [order 2] : [LiquidLevel>=hmax*0.9]
  data: Type input; StartMaintenance input; LiquidIn output; LiquidOut output; LiquidLevel input; hmax parameter

== stateflow chart c00011M_harness/M229/Tank2/Control/Maintenance/Chart ==
  state InitialState
    entry: LiquidIn = 0;
    LiquidOut = 0;
  state Step1
    entry: LiquidIn = 0;
    LiquidOut = 1;
  state Step2
    entry: LiquidIn = 1;
    LiquidOut = 0;
  state Step3
    entry: LiquidIn = 0;
    LiquidOut = 1;
  (default) -> InitialState
  Step3 -> InitialState : [Type~=1||LiquidLevel <=0.01]
  Step2 -> InitialState [order 1] : [Type~=1]
  Step1 -> InitialState [order 1] : [Type ~= 1]
  InitialState -> Step1 : [StartMaintenance == 1 && Type ==1]
  Step1 -> Step2 [order 2] : [LiquidLevel <=0.01]
  Step2 -> Step3 [order 2] : [LiquidLevel>=hmax*0.9]
  data: Type input; StartMaintenance input; LiquidIn output; LiquidOut output; LiquidLevel input; hmax parameter

== stateflow chart c00011M_harness/M230/Tank1/Control/Maintenance/Chart ==
  state InitialState
    entry: LiquidIn = 0;
    LiquidOut = 0;
  state Step1
    entry: LiquidIn = 0;
    LiquidOut = 1;
  state Step2
    entry: LiquidIn = 1;
    LiquidOut = 0;
  state Step3
    entry: LiquidIn = 0;
    LiquidOut = 1;
  (default) -> InitialState
  Step3 -> InitialState : [Type~=1||LiquidLevel <=0.01]
  Step2 -> InitialState [order 1] : [Type~=1]
  Step1 -> InitialState [order 1] : [Type ~= 1]
  InitialState -> Step1 : [StartMaintenance == 1 && Type ==1]
  Step1 -> Step2 [order 2] : [LiquidLevel <=0.01]
  Step2 -> Step3 [order 2] : [LiquidLevel>=hmax*0.9]
  data: Type input; StartMaintenance input; LiquidIn output; LiquidOut output; LiquidLevel input; hmax parameter

== stateflow chart c00011M_harness/M230/Tank2/Control/Maintenance/Chart ==
  state InitialState
    entry: LiquidIn = 0;
    LiquidOut = 0;
  state Step1
    entry: LiquidIn = 0;
    LiquidOut = 1;
  state Step2
    entry: LiquidIn = 1;
    LiquidOut = 0;
  state Step3
    entry: LiquidIn = 0;
    LiquidOut = 1;
  (default) -> InitialState
  Step3 -> InitialState : [Type~=1||LiquidLevel <=0.01]
  Step2 -> InitialState [order 1] : [Type~=1]
  Step1 -> InitialState [order 1] : [Type ~= 1]
  InitialState -> Step1 : [StartMaintenance == 1 && Type ==1]
  Step1 -> Step2 [order 2] : [LiquidLevel <=0.01]
  Step2 -> Step3 [order 2] : [LiquidLevel>=hmax*0.9]
  data: Type input; StartMaintenance input; LiquidIn output; LiquidOut output; LiquidLevel input; hmax parameter

== stateflow chart c00011M_harness/M231/Tank1/Control/Maintenance/Chart ==
  state InitialState
    entry: LiquidIn = 0;
    LiquidOut = 0;
  state Step1
    entry: LiquidIn = 0;
    LiquidOut = 1;
  state Step2
    entry: LiquidIn = 1;
    LiquidOut = 0;
  state Step3
    entry: LiquidIn = 0;
    LiquidOut = 1;
  (default) -> InitialState
  Step3 -> InitialState : [Type~=1||LiquidLevel <=0.01]
  Step2 -> InitialState [order 1] : [Type~=1]
  Step1 -> InitialState [order 1] : [Type ~= 1]
  InitialState -> Step1 : [StartMaintenance == 1 && Type ==1]
  Step1 -> Step2 [order 2] : [LiquidLevel <=0.01]
  Step2 -> Step3 [order 2] : [LiquidLevel>=hmax*0.9]
  data: Type input; StartMaintenance input; LiquidIn output; LiquidOut output; LiquidLevel input; hmax parameter

== stateflow chart c00011M_harness/M231/Tank2/Control/Maintenance/Chart ==
  state InitialState
    entry: LiquidIn = 0;
    LiquidOut = 0;
  state Step1
    entry: LiquidIn = 0;
    LiquidOut = 1;
  state Step2
    entry: LiquidIn = 1;
    LiquidOut = 0;
  state Step3
    entry: LiquidIn = 0;
    LiquidOut = 1;
  (default) -> InitialState
  Step3 -> InitialState : [Type~=1||LiquidLevel <=0.01]
  Step2 -> InitialState [order 1] : [Type~=1]
  Step1 -> InitialState [order 1] : [Type ~= 1]
  InitialState -> Step1 : [StartMaintenance == 1 && Type ==1]
  Step1 -> Step2 [order 2] : [LiquidLevel <=0.01]
  Step2 -> Step3 [order 2] : [LiquidLevel>=hmax*0.9]
  data: Type input; StartMaintenance input; LiquidIn output; LiquidOut output; LiquidLevel input; hmax parameter

== stateflow chart c00011M_harness/M232/Tank1/Control/Maintenance/Chart ==
  state InitialState
    entry: LiquidIn = 0;
    LiquidOut = 0;
  state Step1
    entry: LiquidIn = 0;
    LiquidOut = 1;
  state Step2
    entry: LiquidIn = 1;
    LiquidOut = 0;
  state Step3
    entry: LiquidIn = 0;
    LiquidOut = 1;
  (default) -> InitialState
  Step3 -> InitialState : [Type~=1||LiquidLevel <=0.01]
  Step2 -> InitialState [order 1] : [Type~=1]
  Step1 -> InitialState [order 1] : [Type ~= 1]
  InitialState -> Step1 : [StartMaintenance == 1 && Type ==1]
  Step1 -> Step2 [order 2] : [LiquidLevel <=0.01]
  Step2 -> Step3 [order 2] : [LiquidLevel>=hmax*0.9]
  data: Type input; StartMaintenance input; LiquidIn output; LiquidOut output; LiquidLevel input; hmax parameter

== stateflow chart c00011M_harness/M232/Tank2/Control/Maintenance/Chart ==
  state InitialState
    entry: LiquidIn = 0;
    LiquidOut = 0;
  state Step1
    entry: LiquidIn = 0;
    LiquidOut = 1;
  state Step2
    entry: LiquidIn = 1;
    LiquidOut = 0;
  state Step3
    entry: LiquidIn = 0;
    LiquidOut = 1;
  (default) -> InitialState
  Step3 -> InitialState : [Type~=1||LiquidLevel <=0.01]
  Step2 -> InitialState [order 1] : [Type~=1]
  Step1 -> InitialState [order 1] : [Type ~= 1]
  InitialState -> Step1 : [StartMaintenance == 1 && Type ==1]
  Step1 -> Step2 [order 2] : [LiquidLevel <=0.01]
  Step2 -> Step3 [order 2] : [LiquidLevel>=hmax*0.9]
  data: Type input; StartMaintenance input; LiquidIn output; LiquidOut output; LiquidLevel input; hmax parameter

== stateflow chart c00011M_harness/M233/Tank1/Control/Maintenance/Chart ==
  state InitialState
    entry: LiquidIn = 0;
    LiquidOut = 0;
  state Step1
    entry: LiquidIn = 0;
    LiquidOut = 1;
  state Step2
    entry: LiquidIn = 1;
    LiquidOut = 0;
  state Step3
    entry: LiquidIn = 0;
    LiquidOut = 1;
  (default) -> InitialState
  Step3 -> InitialState : [Type~=1||LiquidLevel <=0.01]
  Step2 -> InitialState [order 1] : [Type~=1]
  Step1 -> InitialState [order 1] : [Type ~= 1]
  InitialState -> Step1 : [StartMaintenance == 1 && Type ==1]
  Step1 -> Step2 [order 2] : [LiquidLevel <=0.01]
  Step2 -> Step3 [order 2] : [LiquidLevel>=hmax*0.9]
  data: Type input; StartMaintenance input; LiquidIn output; LiquidOut output; LiquidLevel input; hmax parameter

== stateflow chart c00011M_harness/M233/Tank2/Control/Maintenance/Chart ==
  state InitialState
    entry: LiquidIn = 0;
    LiquidOut = 0;
  state Step1
    entry: LiquidIn = 0;
    LiquidOut = 1;
  state Step2
    entry: LiquidIn = 1;
    LiquidOut = 0;
  state Step3
    entry: LiquidIn = 0;
    LiquidOut = 1;
  (default) -> InitialState
  Step3 -> InitialState : [Type~=1||LiquidLevel <=0.01]
  Step2 -> InitialState [order 1] : [Type~=1]
  Step1 -> InitialState [order 1] : [Type ~= 1]
  InitialState -> Step1 : [StartMaintenance == 1 && Type ==1]
  Step1 -> Step2 [order 2] : [LiquidLevel <=0.01]
  Step2 -> Step3 [order 2] : [LiquidLevel>=hmax*0.9]
  data: Type input; StartMaintenance input; LiquidIn output; LiquidOut output; LiquidLevel input; hmax parameter

== stateflow chart c00011M_harness/M234/Tank1/Control/Maintenance/Chart ==
  state InitialState
    entry: LiquidIn = 0;
    LiquidOut = 0;
  state Step1
    entry: LiquidIn = 0;
    LiquidOut = 1;
  state Step2
    entry: LiquidIn = 1;
    LiquidOut = 0;
  state Step3
    entry: LiquidIn = 0;
    LiquidOut = 1;
  (default) -> InitialState
  Step3 -> InitialState : [Type~=1||LiquidLevel <=0.01]
  Step2 -> InitialState [order 1] : [Type~=1]
  Step1 -> InitialState [order 1] : [Type ~= 1]
  InitialState -> Step1 : [StartMaintenance == 1 && Type ==1]
  Step1 -> Step2 [order 2] : [LiquidLevel <=0.01]
  Step2 -> Step3 [order 2] : [LiquidLevel>=hmax*0.9]
  data: Type input; StartMaintenance input; LiquidIn output; LiquidOut output; LiquidLevel input; hmax parameter

== stateflow chart c00011M_harness/M234/Tank2/Control/Maintenance/Chart ==
  state InitialState
    entry: LiquidIn = 0;
    LiquidOut = 0;
  state Step1
    entry: LiquidIn = 0;
    LiquidOut = 1;
  state Step2
    entry: LiquidIn = 1;
    LiquidOut = 0;
  state Step3
    entry: LiquidIn = 0;
    LiquidOut = 1;
  (default) -> InitialState
  Step3 -> InitialState : [Type~=1||LiquidLevel <=0.01]
  Step2 -> InitialState [order 1] : [Type~=1]
  Step1 -> InitialState [order 1] : [Type ~= 1]
  InitialState -> Step1 : [StartMaintenance == 1 && Type ==1]
  Step1 -> Step2 [order 2] : [LiquidLevel <=0.01]
  Step2 -> Step3 [order 2] : [LiquidLevel>=hmax*0.9]
  data: Type input; StartMaintenance input; LiquidIn output; LiquidOut output; LiquidLevel input; hmax parameter

== stateflow chart c00011M_harness/M235/Tank1/Control/Maintenance/Chart ==
  state InitialState
    entry: LiquidIn = 0;
    LiquidOut = 0;
  state Step1
    entry: LiquidIn = 0;
    LiquidOut = 1;
  state Step2
    entry: LiquidIn = 1;
    LiquidOut = 0;
  state Step3
    entry: LiquidIn = 0;
    LiquidOut = 1;
  (default) -> InitialState
  Step3 -> InitialState : [Type~=1||LiquidLevel <=0.01]
  Step2 -> InitialState [order 1] : [Type~=1]
  Step1 -> InitialState [order 1] : [Type ~= 1]
  InitialState -> Step1 : [StartMaintenance == 1 && Type ==1]
  Step1 -> Step2 [order 2] : [LiquidLevel <=0.01]
  Step2 -> Step3 [order 2] : [LiquidLevel>=hmax*0.9]
  data: Type input; StartMaintenance input; LiquidIn output; LiquidOut output; LiquidLevel input; hmax parameter

== stateflow chart c00011M_harness/M235/Tank2/Control/Maintenance/Chart ==
  state InitialState
    entry: LiquidIn = 0;
    LiquidOut = 0;
  state Step1
    entry: LiquidIn = 0;
    LiquidOut = 1;
  state Step2
    entry: LiquidIn = 1;
    LiquidOut = 0;
  state Step3
    entry: LiquidIn = 0;
    LiquidOut = 1;
  (default) -> InitialState
  Step3 -> InitialState : [Type~=1||LiquidLevel <=0.01]
  Step2 -> InitialState [order 1] : [Type~=1]
  Step1 -> InitialState [order 1] : [Type ~= 1]
  InitialState -> Step1 : [StartMaintenance == 1 && Type ==1]
  Step1 -> Step2 [order 2] : [LiquidLevel <=0.01]
  Step2 -> Step3 [order 2] : [LiquidLevel>=hmax*0.9]
  data: Type input; StartMaintenance input; LiquidIn output; LiquidOut output; LiquidLevel input; hmax parameter

== stateflow chart c00011M_harness/M236/Tank1/Control/Maintenance/Chart ==
  state InitialState
    entry: LiquidIn = 0;
    LiquidOut = 0;
  state Step1
    entry: LiquidIn = 0;
    LiquidOut = 1;
  state Step2
    entry: LiquidIn = 1;
    LiquidOut = 0;
  state Step3
    entry: LiquidIn = 0;
    LiquidOut = 1;
  (default) -> InitialState
  Step3 -> InitialState : [Type~=1||LiquidLevel <=0.01]
  Step2 -> InitialState [order 1] : [Type~=1]
  Step1 -> InitialState [order 1] : [Type ~= 1]
  InitialState -> Step1 : [StartMaintenance == 1 && Type ==1]
  Step1 -> Step2 [order 2] : [LiquidLevel <=0.01]
  Step2 -> Step3 [order 2] : [LiquidLevel>=hmax*0.9]
  data: Type input; StartMaintenance input; LiquidIn output; LiquidOut output; LiquidLevel input; hmax parameter

== stateflow chart c00011M_harness/M236/Tank2/Control/Maintenance/Chart ==
  state InitialState
    entry: LiquidIn = 0;
    LiquidOut = 0;
  state Step1
    entry: LiquidIn = 0;
    LiquidOut = 1;
  state Step2
    entry: LiquidIn = 1;
    LiquidOut = 0;
  state Step3
    entry: LiquidIn = 0;
    LiquidOut = 1;
  (default) -> InitialState
  Step3 -> InitialState : [Type~=1||LiquidLevel <=0.01]
  Step2 -> InitialState [order 1] : [Type~=1]
  Step1 -> InitialState [order 1] : [Type ~= 1]
  InitialState -> Step1 : [StartMaintenance == 1 && Type ==1]
  Step1 -> Step2 [order 2] : [LiquidLevel <=0.01]
  Step2 -> Step3 [order 2] : [LiquidLevel>=hmax*0.9]
  data: Type input; StartMaintenance input; LiquidIn output; LiquidOut output; LiquidLevel input; hmax parameter

== stateflow chart c00011M_harness/M237/Tank1/Control/Maintenance/Chart ==
  state InitialState
    entry: LiquidIn = 0;
    LiquidOut = 0;
  state Step1
    entry: LiquidIn = 0;
    LiquidOut = 1;
  state Step2
    entry: LiquidIn = 1;
    LiquidOut = 0;
  state Step3
    entry: LiquidIn = 0;
    LiquidOut = 1;
  (default) -> InitialState
  Step3 -> InitialState : [Type~=1||LiquidLevel <=0.01]
  Step2 -> InitialState [order 1] : [Type~=1]
  Step1 -> InitialState [order 1] : [Type ~= 1]
  InitialState -> Step1 : [StartMaintenance == 1 && Type ==1]
  Step1 -> Step2 [order 2] : [LiquidLevel <=0.01]
  Step2 -> Step3 [order 2] : [LiquidLevel>=hmax*0.9]
  data: Type input; StartMaintenance input; LiquidIn output; LiquidOut output; LiquidLevel input; hmax parameter

== stateflow chart c00011M_harness/M237/Tank2/Control/Maintenance/Chart ==
  state InitialState
    entry: LiquidIn = 0;
    LiquidOut = 0;
  state Step1
    entry: LiquidIn = 0;
    LiquidOut = 1;
  state Step2
    entry: LiquidIn = 1;
    LiquidOut = 0;
  state Step3
    entry: LiquidIn = 0;
    LiquidOut = 1;
  (default) -> InitialState
  Step3 -> InitialState : [Type~=1||LiquidLevel <=0.01]
  Step2 -> InitialState [order 1] : [Type~=1]
  Step1 -> InitialState [order 1] : [Type ~= 1]
  InitialState -> Step1 : [StartMaintenance == 1 && Type ==1]
  Step1 -> Step2 [order 2] : [LiquidLevel <=0.01]
  Step2 -> Step3 [order 2] : [LiquidLevel>=hmax*0.9]
  data: Type input; StartMaintenance input; LiquidIn output; LiquidOut output; LiquidLevel input; hmax parameter

== stateflow chart c00011M_harness/M238/Tank1/Control/Maintenance/Chart ==
  state InitialState
    entry: LiquidIn = 0;
    LiquidOut = 0;
  state Step1
    entry: LiquidIn = 0;
    LiquidOut = 1;
  state Step2
    entry: LiquidIn = 1;
    LiquidOut = 0;
  state Step3
    entry: LiquidIn = 0;
    LiquidOut = 1;
  (default) -> InitialState
  Step3 -> InitialState : [Type~=1||LiquidLevel <=0.01]
  Step2 -> InitialState [order 1] : [Type~=1]
  Step1 -> InitialState [order 1] : [Type ~= 1]
  InitialState -> Step1 : [StartMaintenance == 1 && Type ==1]
  Step1 -> Step2 [order 2] : [LiquidLevel <=0.01]
  Step2 -> Step3 [order 2] : [LiquidLevel>=hmax*0.9]
  data: Type input; StartMaintenance input; LiquidIn output; LiquidOut output; LiquidLevel input; hmax parameter

== stateflow chart c00011M_harness/M238/Tank2/Control/Maintenance/Chart ==
  state InitialState
    entry: LiquidIn = 0;
    LiquidOut = 0;
  state Step1
    entry: LiquidIn = 0;
    LiquidOut = 1;
  state Step2
    entry: LiquidIn = 1;
    LiquidOut = 0;
  state Step3
    entry: LiquidIn = 0;
    LiquidOut = 1;
  (default) -> InitialState
  Step3 -> InitialState : [Type~=1||LiquidLevel <=0.01]
  Step2 -> InitialState [order 1] : [Type~=1]
  Step1 -> InitialState [order 1] : [Type ~= 1]
  InitialState -> Step1 : [StartMaintenance == 1 && Type ==1]
  Step1 -> Step2 [order 2] : [LiquidLevel <=0.01]
  Step2 -> Step3 [order 2] : [LiquidLevel>=hmax*0.9]
  data: Type input; StartMaintenance input; LiquidIn output; LiquidOut output; LiquidLevel input; hmax parameter

== stateflow chart c00011M_harness/M239/Tank1/Control/Maintenance/Chart ==
  state InitialState
    entry: LiquidIn = 0;
    LiquidOut = 0;
  state Step1
    entry: LiquidIn = 0;
    LiquidOut = 1;
  state Step2
    entry: LiquidIn = 1;
    LiquidOut = 0;
  state Step3
    entry: LiquidIn = 0;
    LiquidOut = 1;
  (default) -> InitialState
  Step3 -> InitialState : [Type~=1||LiquidLevel <=0.01]
  Step2 -> InitialState [order 1] : [Type~=1]
  Step1 -> InitialState [order 1] : [Type ~= 1]
  InitialState -> Step1 : [StartMaintenance == 1 && Type ==1]
  Step1 -> Step2 [order 2] : [LiquidLevel <=0.01]
  Step2 -> Step3 [order 2] : [LiquidLevel>=hmax*0.9]
  data: Type input; StartMaintenance input; LiquidIn output; LiquidOut output; LiquidLevel input; hmax parameter

== stateflow chart c00011M_harness/M239/Tank2/Control/Maintenance/Chart ==
  state InitialState
    entry: LiquidIn = 0;
    LiquidOut = 0;
  state Step1
    entry: LiquidIn = 0;
    LiquidOut = 1;
  state Step2
    entry: LiquidIn = 1;
    LiquidOut = 0;
  state Step3
    entry: LiquidIn = 0;
    LiquidOut = 1;
  (default) -> InitialState
  Step3 -> InitialState : [Type~=1||LiquidLevel <=0.01]
  Step2 -> InitialState [order 1] : [Type~=1]
  Step1 -> InitialState [order 1] : [Type ~= 1]
  InitialState -> Step1 : [StartMaintenance == 1 && Type ==1]
  Step1 -> Step2 [order 2] : [LiquidLevel <=0.01]
  Step2 -> Step3 [order 2] : [LiquidLevel>=hmax*0.9]
  data: Type input; StartMaintenance input; LiquidIn output; LiquidOut output; LiquidLevel input; hmax parameter
